simulink model "MotorVCUs_v1"  (R2019b)
settings: Solver=VariableStepAuto  StartTime=0.0  StopTime=10.0  RelTol=1e-3

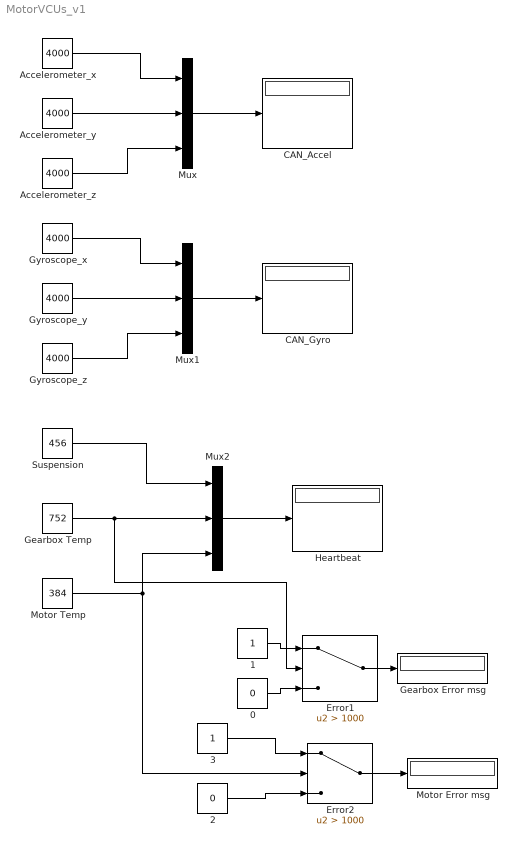
== system MotorVCUs_v1 ==
  0 : Constant  Value=0
  1 : Constant
  2 : Constant  Value=0
  3 : Constant
  Accelerometer_x : Constant  Value=4000
  Accelerometer_y : Constant  Value=4000
  Accelerometer_z : Constant  Value=4000
  CAN_Accel : Display
  CAN_Gyro : Display
  Error1 : Switch  Criteria=u2 > Threshold  Threshold=1000
  Error2 : Switch  Criteria=u2 > Threshold  Threshold=1000
  Gearbox Error msg : Display
  Gearbox Temp : Constant  Value=752
  Gyroscope_x : Constant  Value=4000
  Gyroscope_y : Constant  Value=4000
  Gyroscope_z : Constant  Value=4000
  Heartbeat : Display
  Motor Error msg : Display
  Motor Temp : Constant  Value=384
  Mux : Mux  Inputs=3
  Mux1 : Mux  Inputs=3
  Mux2 : Mux  Inputs=3
  Suspension : Constant  Value=456
  wires:
  Accelerometer_x/1 -> Mux/1
  Accelerometer_y/1 -> Mux/2
  Accelerometer_z/1 -> Mux/3
  Mux/1 -> CAN_Accel/1
  Gyroscope_y/1 -> Mux1/2
  Gyroscope_z/1 -> Mux1/3
  Gyroscope_x/1 -> Mux1/1
  Mux1/1 -> CAN_Gyro/1
  Gearbox Temp/1 -> Error1/2, Mux2/2
  Suspension/1 -> Mux2/1
  Mux2/1 -> Heartbeat/1
  0/1 -> Error1/3
  1/1 -> Error1/1
  2/1 -> Error2/3
  Motor Temp/1 -> Error2/2, Mux2/3
  3/1 -> Error2/1
  Error1/1 -> Gearbox Error msg/1
  Error2/1 -> Motor Error msg/1
